simulink model "uz_6ph_pu_voltages_vsd"  (R2021a)
settings: Solver=FixedStepDiscrete  StartTime=0.0  StopTime=1/f  RelTol=1e-3
values from neighbouring files (symbols this model uses):
  f = n_rpm/60.0*p    (= 250)    [uz_6ph_pu_voltages_vsd_init.m]
  t_ADC = 1/f_ADC    (= 1e-05)    [uz_6ph_pu_voltages_vsd_init.m]
  v_dc = 565.0    (= 565)    [uz_6ph_pu_voltages_vsd_init.m]
  VB = sqrt(2/3)*VR    [uz_6ph_pu_voltages_vsd_init.m]
libraries: simulink x2, hdlsllib x1
settings Model: DataTypeOverride=Off  Creator=micha  LastModifiedBy=micha
settings SolverCC: AlgebraicLoopSolver=TrustRegion
settings DataIOCC: LimitDataPoints=on  SaveOutput=off  SaveTime=off
settings OptimizationCC: BlockReduction=off  ConditionallyExecuteInputs=off  DefaultParameterBehavior=Inlined  ExpressionDepthLimit=2147483647  InitFltsAndDblsToZero=on  LifeSpan=inf
settings DebuggingCC: AlgebraicLoopMsg=error  UnderspecifiedInitializationDetection=Classic  MergeDetectMultiDrivingBlocksExec=none  SingleTaskRateTransMsg=error  FcnCallInpInsideContextMsg=warning  AllowSymbolicDim=off  StateNameClashWarn=warning  StrictBusMsg=ErrorOnBusTreatedAsVector  SFUnexpectedBacktrackingDiag=warning  SFNoUnconditionalDefaultTransitionDiag=warning  SFExecutionAtInitializationDiag=none  SFMachineParentedDataDiag=warning  ArithmeticOperatorsInVariantConditions=warning
settings HardwareCC: ProdBitPerPointer=32  ProdBitPerSizeT=32  ProdBitPerPtrDiffT=32  ProdLargestAtomicFloat=None  ProdIntDivRoundTo=Undefined  ProdEndianess=Unspecified  ProdWordSize=32  ProdHWDeviceType=ASIC/FPGA->ASIC/FPGA  ProdEqTarget=off
settings SFSimCC: SimUseLocalCustomCode=off  SimParseCustomCode=off  CustomCodeUndefinedFunction=UseInterfaceOnly
settings RTWCC: RTWUseLocalCustomCode=off
settings CodeAppCC: StateflowObjectComments=on
settings GRTTargetCC: TargetLangStandard=C89/C90 (ANSI)  CombineOutputUpdateFcns=off  GRTInterface=on
settings ConfigComp: CovScope=ReferencedModels  CovMetricSettings=dw  CovSaveCumulativeToWorkspaceVar=on  CovSaveSingleToWorkspaceVar=on  CovExternalEMLEnable=off  CovSFcnEnable=off

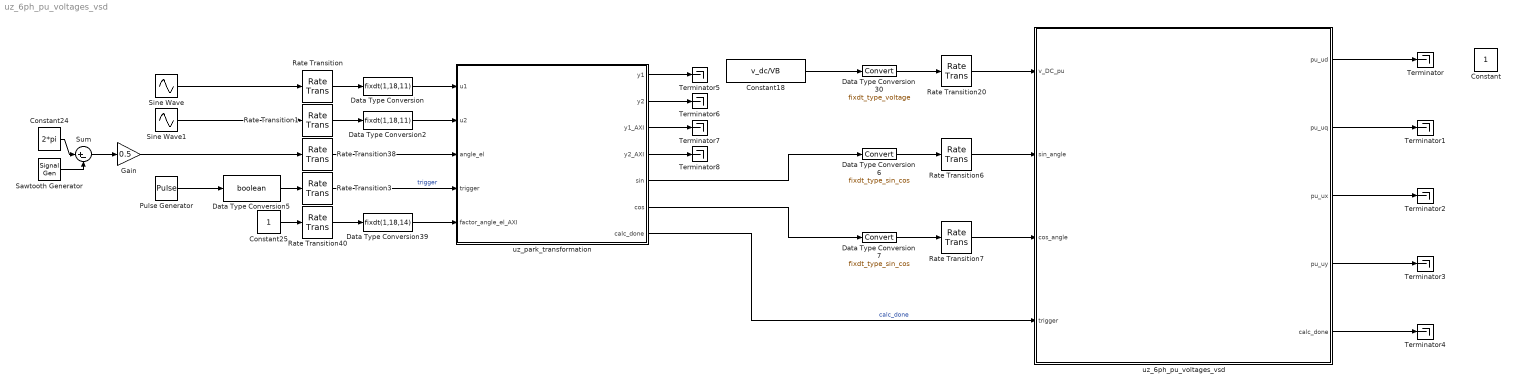
== system uz_6ph_pu_voltages_vsd ==
  Constant : Constant
  Constant18 : Constant  Value=v_dc/VB
  Constant24 : Constant  Value=2*pi
  Constant25 : Constant
  Data Type Conversion : DataTypeConversion  OutDataTypeStr=fixdt(1,18,11)
  Data Type Conversion2 : DataTypeConversion  OutDataTypeStr=fixdt(1,18,11)
  Data Type Conversion30 : DataTypeConversion  OutDataTypeStr=fixdt_type_voltage
  Data Type Conversion39 : DataTypeConversion  OutDataTypeStr=fixdt(1,18,14)
  Data Type Conversion5 : DataTypeConversion  OutDataTypeStr=boolean
  Data Type Conversion6 : DataTypeConversion  OutDataTypeStr=fixdt_type_sin_cos
  Data Type Conversion7 : DataTypeConversion  OutDataTypeStr=fixdt_type_sin_cos
  Gain : Gain  Gain=0.5
  Pulse Generator : DiscretePulseGenerator  PulseType=Time based  Period=t_ADC  PulseWidth=5
  Rate Transition{,1,3,6..7,20,38,40} (8 alike) : RateTransition  OutPortSampleTime=t_clock
  Sawtooth Generator : SignalGenerator  WaveForm=sawtooth  Amplitude=2*pi  Frequency=2*pi*f  Units=rad/sec
  Sine Wave : Sin  Frequency=2*pi*f  SampleTime=0
  Sine Wave1 : Sin  Frequency=2*pi*f  Phase=-pi/2  SampleTime=0
  Sum : Sum  Inputs=|+-
  Terminator{,1..8} (9 alike) : Terminator
  uz_6ph_pu_voltages_vsd : Subsystem
  uz_park_transformation : Subsystem  TreatAsAtomicUnit=on
  wires:
  Data Type Conversion30/1 -> Rate Transition20/1
  Rate Transition20/1 -> uz_6ph_pu_voltages_vsd/1(v_DC_pu)
  Constant18/1 -> Data Type Conversion30/1
  Data Type Conversion6/1 -> Rate Transition6/1
  Rate Transition7/1 -> uz_6ph_pu_voltages_vsd/3(cos_angle)
  Rate Transition6/1 -> uz_6ph_pu_voltages_vsd/2(sin_angle)
  Data Type Conversion7/1 -> Rate Transition7/1
  Constant25/1 -> Rate Transition40/1
  Rate Transition40/1 -> Data Type Conversion39/1
  uz_park_transformation/7(calc_done) -> uz_6ph_pu_voltages_vsd/4(trigger)  "calc_done"
  Sawtooth Generator/1 -> Sum/2
  Data Type Conversion39/1 -> uz_park_transformation/5(factor_angle_el_AXI)
  Gain/1 -> Rate Transition38/1
  Sum/1 -> Gain/1
  Constant24/1 -> Sum/1
  Rate Transition38/1 -> uz_park_transformation/3(angle_el)
  uz_park_transformation/5(sin) -> Data Type Conversion6/1
  uz_park_transformation/6(cos) -> Data Type Conversion7/1
  Rate Transition1/1 -> Data Type Conversion2/1
  Rate Transition/1 -> Data Type Conversion/1
  Sine Wave/1 -> Rate Transition/1
  Sine Wave1/1 -> Rate Transition1/1
  Data Type Conversion/1 -> uz_park_transformation/1(u1)
  Data Type Conversion2/1 -> uz_park_transformation/2(u2)
  Data Type Conversion5/1 -> Rate Transition3/1
  Pulse Generator/1 -> Data Type Conversion5/1
  Rate Transition3/1 -> uz_park_transformation/4(trigger)  "trigger"
  uz_6ph_pu_voltages_vsd/1(pu_ud) -> Terminator/1
  uz_6ph_pu_voltages_vsd/2(pu_uq) -> Terminator1/1
  uz_6ph_pu_voltages_vsd/3(pu_ux) -> Terminator2/1
  uz_6ph_pu_voltages_vsd/4(pu_uy) -> Terminator3/1
  uz_6ph_pu_voltages_vsd/5(calc_done) -> Terminator4/1
  uz_park_transformation/1(y1) -> Terminator5/1
  uz_park_transformation/2(y2) -> Terminator6/1
  uz_park_transformation/3(y1_AXI) -> Terminator7/1
  uz_park_transformation/4(y2_AXI) -> Terminator8/1

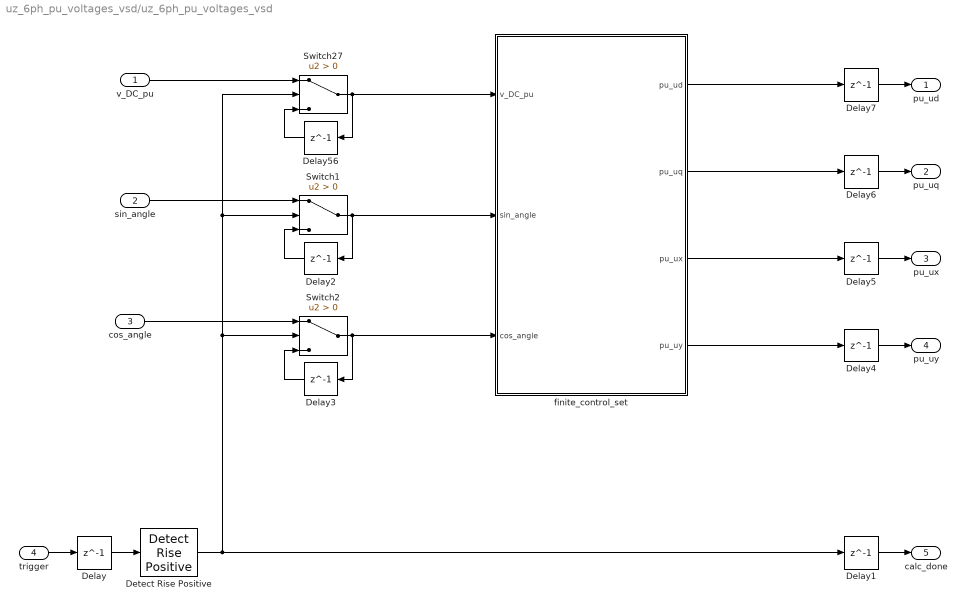
== system uz_6ph_pu_voltages_vsd/uz_6ph_pu_voltages_vsd ==
  v_DC_pu : Inport
  sin_angle : Inport  Port=2
  cos_angle : Inport  Port=3
  trigger : Inport  Port=4
  Delay{,1..7,56} (9 alike) : Delay  DelayLength=1
  Detect Rise Positive : simulink/Logic and Bit Operations/Detect Rise Positive  vinit=0  OutDataTypeStr=boolean
  Switch1 : Switch  Criteria=u2 > Threshold
  Switch2 : Switch  Criteria=u2 > Threshold
  Switch27 : Switch  Criteria=u2 > Threshold
  finite_control_set : MATLAB Function  TreatAsAtomicUnit=on
  pu_ud : Outport
  pu_uq : Outport  Port=2
  pu_ux : Outport  Port=3
  pu_uy : Outport  Port=4
  calc_done : Outport  Port=5
  wires:
  finite_control_set/1(pu_ud) -> Delay7/1
  finite_control_set/2(pu_uq) -> Delay6/1
  finite_control_set/3(pu_ux) -> Delay5/1
  finite_control_set/4(pu_uy) -> Delay4/1
  trigger/1 -> Delay/1
  Delay/1 -> Detect Rise Positive/1
  Delay1/1 -> calc_done/1
  Delay56/1 -> Switch27/3
  v_DC_pu/1 -> Switch27/1
  Switch27/1 -> Delay56/1, finite_control_set/1(v_DC_pu)
  sin_angle/1 -> Switch1/1
  Delay2/1 -> Switch1/3
  Switch1/1 -> finite_control_set/2(sin_angle), Delay2/1
  cos_angle/1 -> Switch2/1
  Delay3/1 -> Switch2/3
  Switch2/1 -> finite_control_set/3(cos_angle), Delay3/1
  Detect Rise Positive/1 -> Switch2/2, Switch1/2, Switch27/2, Delay1/1
  Delay4/1 -> pu_uy/1
  Delay5/1 -> pu_ux/1
  Delay6/1 -> pu_uq/1
  Delay7/1 -> pu_ud/1

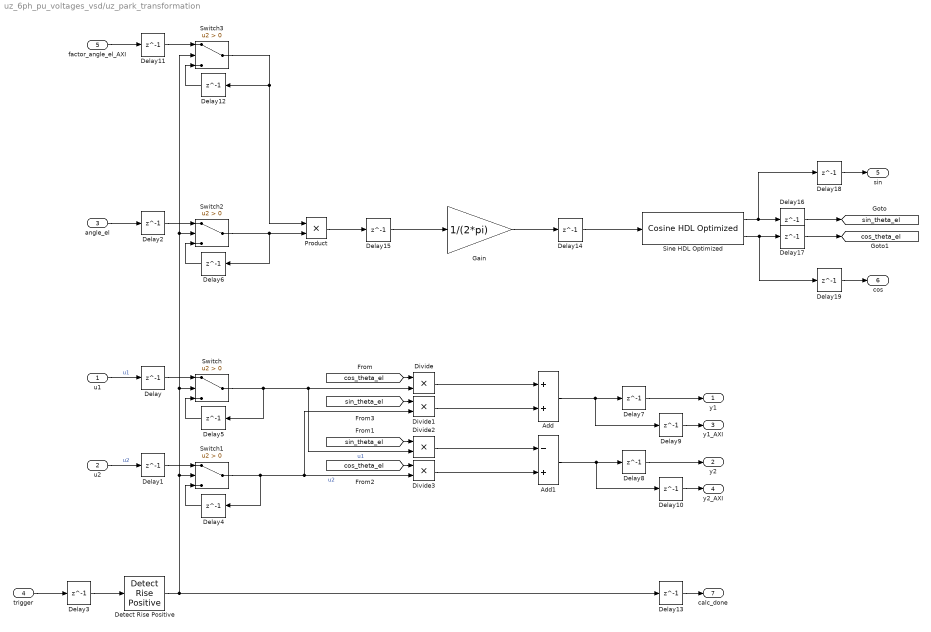
== system uz_6ph_pu_voltages_vsd/uz_park_transformation ==
  u1 : Inport
  u2 : Inport  Port=2
  angle_el : Inport  Port=3
  trigger : Inport  Port=4
  factor_angle_el_AXI : Inport  Port=5
  Add : Sum  OutDataTypeStr=fixdt(1,27,16)
  Add1 : Sum  Inputs=-+  OutDataTypeStr=fixdt(1,27,16)
  Delay{,1..19} (20 alike) : Delay  DelayLength=1
  Detect Rise Positive : simulink/Logic and Bit Operations/Detect Rise Positive  vinit=0  OutDataTypeStr=boolean
  Divide{,1..3} (4 alike) : Product  Inputs=**  OutDataTypeStr=fixdt(1,27,16)
  Gain : Gain  Gain=1/(2*pi)  OutDataTypeStr=fixdt(1,18,16)
  Product : Product  OutDataTypeStr=fixdt(1,18,14)
  Sine HDL Optimized : hdlsllib/Lookup Tables/Cosine HDL Optimized  OutputFormula=sin(2*pi*u) and cos(2*pi*u)  NumDataPoints=256  TableDataTypeStr=fixdt(0,17,16)  SimulateLUTROMDelay=off
      settings: SourceProductBaseCode=SL
  Switch{,1..3} (4 alike) : Switch  Criteria=u2 > Threshold
  y1 : Outport  VectorParamsAs1DForOutWhenUnconnected=off
  y2 : Outport  Port=2  VectorParamsAs1DForOutWhenUnconnected=off
  y1_AXI : Outport  Port=3  VectorParamsAs1DForOutWhenUnconnected=off
  y2_AXI : Outport  Port=4  VectorParamsAs1DForOutWhenUnconnected=off
  sin : Outport  Port=5  VectorParamsAs1DForOutWhenUnconnected=off
  cos : Outport  Port=6  VectorParamsAs1DForOutWhenUnconnected=off
  calc_done : Outport  Port=7  VectorParamsAs1DForOutWhenUnconnected=off
  tag scope: cos_theta_el=global, sin_theta_el=global
  wires:
  Switch1/1 -> Delay4/1, Divide1/2, Divide3/2  "u2"
  Divide2/1 -> Add1/1
  Divide3/1 -> Add1/2
  [cos_theta_el] -> Divide3/1
  Switch/1 -> Divide2/2, Divide/2, Delay5/1  "u1"
  [sin_theta_el] -> Divide2/1
  Divide1/1 -> Add/2
  [cos_theta_el] -> Divide/1
  [sin_theta_el] -> Divide1/1
  Add/1 -> Delay9/1, Delay7/1
  Add1/1 -> Delay10/1, Delay8/1
  Divide/1 -> Add/1
  angle_el/1 -> Delay2/1
  Sine HDL Optimized/2 -> Delay19/1, Delay17/1
  Sine HDL Optimized/1 -> Delay18/1, Delay16/1
  Gain/1 -> Delay14/1
  u1/1 -> Delay/1  "u1"
  u2/1 -> Delay1/1  "u2"
  Delay/1 -> Switch/1
  Delay1/1 -> Switch1/1
  Delay2/1 -> Switch2/1
  trigger/1 -> Delay3/1
  Delay4/1 -> Switch1/3
  Delay5/1 -> Switch/3
  Delay6/1 -> Switch2/3
  Delay7/1 -> y1/1
  Delay8/1 -> y2/1
  Delay9/1 -> y1_AXI/1
  Delay10/1 -> y2_AXI/1
  Switch2/1 -> Product/2, Delay6/1
  Switch3/1 -> Product/1, Delay12/1
  factor_angle_el_AXI/1 -> Delay11/1
  Detect Rise Positive/1 -> Delay13/1, Switch1/2, Switch/2, Switch3/2, Switch2/2
  Delay12/1 -> Switch3/3
  Delay11/1 -> Switch3/1
  Product/1 -> Delay15/1
  Delay3/1 -> Detect Rise Positive/1
  Delay13/1 -> calc_done/1
  Delay15/1 -> Gain/1
  Delay14/1 -> Sine HDL Optimized/1
  Delay16/1 -> [sin_theta_el]
  Delay17/1 -> [cos_theta_el]
  Delay18/1 -> sin/1
  Delay19/1 -> cos/1

== matlab function uz_6ph_pu_voltages_vsd/finite_control_set ==
  data: v_DC_pu input; sin_angle input; pu_ud output; pu_uq output; pu_ux output; pu_uy output; cos_angle input
function [pu_ud,pu_uq,pu_ux,pu_uy] = voltage_space_vectors(v_DC_pu, sin_angle, cos_angle)
                          
% u_d-voltages
vd_pu = v_DC_pu * fi([0.000000*cos_angle + 0.000000*sin_angle;
0.333333*cos_angle + -0.000000*sin_angle;
-0.166667*cos_angle + 0.288675*sin_angle;
0.166667*cos_angle + 0.288675*sin_angle;
-0.166667*cos_angle + -0.288675*sin_angle;
0.166667*cos_angle + -0.288675*sin_angle;
-0.333333*cos_angle + 0.000000*sin_angle;
0.000000*cos_angle + 0.000000*sin_angle;
0.288675*cos_angle + 0.166667*sin_angle;
0.622008*cos_angle + 0.166667*sin_angle;
0.122008*cos_angle + 0.455342*sin_angle;
0.455342*cos_angle + 0.455342*sin_angle;
0.122008*cos_angle + -0.122008*sin_angle;
0.455342*cos_angle + -0.122008*sin_angle;
-0.044658*cos_angle + 0.166667*sin_angle;
0.288675*cos_angle + 0.166667*sin_angle;
-0.288675*cos_angle + 0.166667*sin_angle;
0.044658*cos_angle + 0.166667*sin_angle;
-0.455342*cos_angle + 0.455342*sin_angle;
-0.122008*cos_angle + 0.455342*sin_angle;
-0.455342*cos_angle + -0.122008*sin_angle;
-0.122008*cos_angle + -0.122008*sin_angle;
-0.622008*cos_angle + 0.166667*sin_angle;
-0.288675*cos_angle + 0.166667*sin_angle;
0.000000*cos_angle + 0.333333*sin_angle;
0.333333*cos_angle + 0.333333*sin_angle;
-0.166667*cos_angle + 0.622008*sin_angle;
0.166667*cos_angle + 0.622008*sin_angle;
-0.166667*cos_angle + 0.044658*sin_angle;
0.166667*cos_angle + 0.044658*sin_angle;
-0.333333*cos_angle + 0.333333*sin_angle;
0.000000*cos_angle + 0.333333*sin_angle;
-0.000000*cos_angle + -0.333333*sin_angle;
0.333333*cos_angle + -0.333333*sin_angle;
-0.166667*cos_angle + -0.044658*sin_angle;
0.166667*cos_angle + -0.044658*sin_angle;
-0.166667*cos_angle + -0.622008*sin_angle;
0.166667*cos_angle + -0.622008*sin_angle;
-0.333333*cos_angle + -0.333333*sin_angle;
-0.000000*cos_angle + -0.333333*sin_angle;
0.288675*cos_angle + -0.166667*sin_angle;
0.622008*cos_angle + -0.166667*sin_angle;
0.122008*cos_angle + 0.122008*sin_angle;
0.455342*cos_angle + 0.122008*sin_angle;
0.122008*cos_angle + -0.455342*sin_angle;
0.455342*cos_angle + -0.455342*sin_angle;
-0.044658*cos_angle + -0.166667*sin_angle;
0.288675*cos_angle + -0.166667*sin_angle;
-0.288675*cos_angle + -0.166667*sin_angle;
0.044658*cos_angle + -0.166667*sin_angle;
-0.455342*cos_angle + 0.122008*sin_angle;
-0.122008*cos_angle + 0.122008*sin_angle;
-0.455342*cos_angle + -0.455342*sin_angle;
-0.122008*cos_angle + -0.455342*sin_angle;
-0.622008*cos_angle + -0.166667*sin_angle;
-0.288675*cos_angle + -0.166667*sin_angle;
0.000000*cos_angle + 0.000000*sin_angle;
0.333333*cos_angle + -0.000000*sin_angle;
-0.166667*cos_angle + 0.288675*sin_angle;
0.166667*cos_angle + 0.288675*sin_angle;
-0.166667*cos_angle + -0.288675*sin_angle;
0.166667*cos_angle + -0.288675*sin_angle;
-0.333333*cos_angle + 0.000000*sin_angle;
0.000000*cos_angle + 0.000000*sin_angle],1,18,15);

% u_q-voltages
vq_pu = v_DC_pu * fi([0.000000*-sin_angle + 0.000000*cos_angle;
0.333333*-sin_angle + -0.000000*cos_angle;
-0.166667*-sin_angle + 0.288675*cos_angle;
0.166667*-sin_angle + 0.288675*cos_angle;
-0.166667*-sin_angle + -0.288675*cos_angle;
0.166667*-sin_angle + -0.288675*cos_angle;
-0.333333*-sin_angle + 0.000000*cos_angle;
0.000000*-sin_angle + 0.000000*cos_angle;
0.288675*-sin_angle + 0.166667*cos_angle;
0.622008*-sin_angle + 0.166667*cos_angle;
0.122008*-sin_angle + 0.455342*cos_angle;
0.455342*-sin_angle + 0.455342*cos_angle;
0.122008*-sin_angle + -0.122008*cos_angle;
0.455342*-sin_angle + -0.122008*cos_angle;
-0.044658*-sin_angle + 0.166667*cos_angle;
0.288675*-sin_angle + 0.166667*cos_angle;
-0.288675*-sin_angle + 0.166667*cos_angle;
0.044658*-sin_angle + 0.166667*cos_angle;
-0.455342*-sin_angle + 0.455342*cos_angle;
-0.122008*-sin_angle + 0.455342*cos_angle;
-0.455342*-sin_angle + -0.122008*cos_angle;
-0.122008*-sin_angle + -0.122008*cos_angle;
-0.622008*-sin_angle + 0.166667*cos_angle;
-0.288675*-sin_angle + 0.166667*cos_angle;
0.000000*-sin_angle + 0.333333*cos_angle;
0.333333*-sin_angle + 0.333333*cos_angle;
-0.166667*-sin_angle + 0.622008*cos_angle;
0.166667*-sin_angle + 0.622008*cos_angle;
-0.166667*-sin_angle + 0.044658*cos_angle;
0.166667*-sin_angle + 0.044658*cos_angle;
-0.333333*-sin_angle + 0.333333*cos_angle;
0.000000*-sin_angle + 0.333333*cos_angle;
-0.000000*-sin_angle + -0.333333*cos_angle;
0.333333*-sin_angle + -0.333333*cos_angle;
-0.166667*-sin_angle + -0.044658*cos_angle;
0.166667*-sin_angle + -0.044658*cos_angle;
-0.166667*-sin_angle + -0.622008*cos_angle;
0.166667*-sin_angle + -0.622008*cos_angle;
-0.333333*-sin_angle + -0.333333*cos_angle;
-0.000000*-sin_angle + -0.333333*cos_angle;
0.288675*-sin_angle + -0.166667*cos_angle;
0.622008*-sin_angle + -0.166667*cos_angle;
0.122008*-sin_angle + 0.122008*cos_angle;
0.455342*-sin_angle + 0.122008*cos_angle;
0.122008*-sin_angle + -0.455342*cos_angle;
0.455342*-sin_angle + -0.455342*cos_angle;
-0.044658*-sin_angle + -0.166667*cos_angle;
0.288675*-sin_angle + -0.166667*cos_angle;
-0.288675*-sin_angle + -0.166667*cos_angle;
0.044658*-sin_angle + -0.166667*cos_angle;
-0.455342*-sin_angle + 0.122008*cos_angle;
-0.122008*-sin_angle + 0.122008*cos_angle;
-0.455342*-sin_angle + -0.455342*cos_angle;
-0.122008*-sin_angle + -0.455342*cos_angle;
-0.622008*-sin_angle + -0.166667*cos_angle;
-0.288675*-sin_angle + -0.166667*cos_angle;
0.000000*-sin_angle + 0.000000*cos_angle;
0.333333*-sin_angle + -0.000000*cos_angle;
-0.166667*-sin_angle + 0.288675*cos_angle;
0.166667*-sin_angle + 0.288675*cos_angle;
-0.166667*-sin_angle + -0.288675*cos_angle;
0.166667*-sin_angle + -0.288675*cos_angle;
-0.333333*-sin_angle + 0.000000*cos_angle;
0.000000*-sin_angle + 0.000000*cos_angle],1,18,15);
     
% u_x-voltages
vx_pu = v_DC_pu * fi([0.000000;
0.333333;
-0.166667;
0.166667;
-0.166667;
0.166667;
-0.333333;
0.000000;
-0.288675;
0.044658;
-0.455342;
-0.122008;
-0.455342;
-0.122008;
-0.622008;
-0.288675;
0.288675;
0.622008;
0.122008;
0.455342;
0.122008;
0.455342;
-0.044658;
0.288675;
0.000000;
0.333333;
-0.166667;
0.166667;
-0.166667;
0.166667;
-0.333333;
0.000000;
-0.000000;
0.333333;
-0.166667;
0.166667;
-0.166667;
0.166667;
-0.333333;
-0.000000;
-0.288675;
0.044658;
-0.455342;
-0.122008;
-0.455342;
-0.122008;
-0.622008;
-0.288675;
0.288675;
0.622008;
0.122008;
0.455342;
0.122008;
0.455342;
-0.044658;
0.288675;
0.000000;
0.333333;
-0.166667;
0.166667;
-0.166667;
0.166667;
-0.333333;
0.000000],1,18,15);

% u_y-voltages
vy_pu = v_DC_pu * fi([0.000000;
-0.000000;
-0.288675;
-0.288675;
0.288675;
0.288675;
0.000000;
0.000000;
0.166667;
0.166667;
-0.122008;
-0.122008;
0.455342;
0.455342;
0.166667;
0.166667;
0.166667;
0.166667;
-0.122008;
-0.122008;
0.455342;
0.455342;
0.166667;
0.166667;
0.333333;
0.333333;
0.044658;
0.044658;
0.622008;
0.622008;
0.333333;
0.333333;
-0.333333;
-0.333333;
-0.622008;
-0.622008;
-0.044658;
-0.044658;
-0.333333;
-0.333333;
-0.166667;
-0.166667;
-0.455342;
-0.455342;
0.122008;
0.122008;
-0.166667;
-0.166667;
-0.166667;
-0.166667;
-0.455342;
-0.455342;
0.122008;
0.122008;
-0.166667;
-0.166667;
0.000000;
-0.000000;
-0.288675;
-0.288675;
0.288675;
0.288675;
0.000000;
0.000000],1,18,15);

pu_ud = fi(vd_pu,1,27,24);
pu_uq = fi(vq_pu,1,27,24);
pu_ux = fi(vx_pu,1,27,24);
pu_uy = fi(vy_pu,1,27,24);
